simulink model "ACCBase001"  (Simulink 8.3)
settings: Solver=FixedStepDiscrete  StartTime=0.0  StopTime=10.0  FixedStep=0.1  RelTol=1e-3
model workspace (MAT data in the model file):
  pACC.Kp = 0.1
  pACC.minDist2Target = 50
  pACC.Ki = 0.0001
  pACC.KpDist = 1
  pACC.KiDist = 0.0001
  MPS_ModuleName = 'ACC_Enhancement.ECR'
settings Model: Creator=swami  LastModifiedBy=swami
settings DataIOCC: SignalLoggingSaveFormat=Dataset
settings DebuggingCC: UnderspecifiedInitializationDetection=Simplified  StateNameClashWarn=none
settings GRTTargetCC: CombineOutputUpdateFcns=on  GRTInterface=off

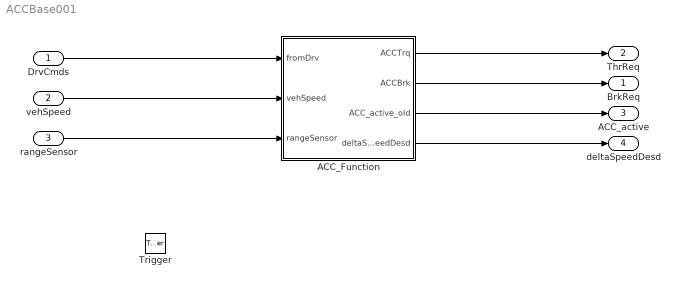
== system ACCBase001 ==
  DrvCmds : Inport  PortDimensions=4
  vehSpeed : Inport  Port=2
  rangeSensor : Inport  Port=3
  Trigger : TriggerPort  TriggerType=function-call  PortDimensions=1
  ACC_Function : MATLAB Function  TreatAsAtomicUnit=on
  BrkReq : Outport  PortDimensions=1
  ThrReq : Outport  Port=2  PortDimensions=1
  ACC_active : Outport  Port=3  PortDimensions=1
  deltaSpeedDesd : Outport  Port=4  PortDimensions=1
  wires:
  DrvCmds/1 -> ACC_Function/1(fromDrv)
  ACC_Function/1(ACCTrq) -> ThrReq/1
  ACC_Function/2(ACCBrk) -> BrkReq/1
  rangeSensor/1 -> ACC_Function/3(rangeSensor)
  vehSpeed/1 -> ACC_Function/2(vehSpeed)
  ACC_Function/3(ACC_active_old) -> ACC_active/1
  ACC_Function/4(deltaSpeedDesd) -> deltaSpeedDesd/1

== matlab function ACC_Function ==
  data: fromDrv input double; ACCTrq output double; ACCBrk output double; vehSpeed input double; rangeSensor input double; pACC parameter double; ACC_active_old output double; deltaSpeedDesd output double
function [ACCTrq,ACCBrk,ACC_active_old,deltaSpeedDesd] = fcn(fromDrv,vehSpeed,rangeSensor,pACC)
%#codegen
persistent dbgcnt;
persistent CC_active;
persistent ACC_active;
persistent torq_req_int;
persistent torq_req_old;
persistent errorKiDist;
if isempty(ACC_active)
    CC_active = 0;
    ACC_active = 0;
    torq_req_int = 0;
    torq_req_old = 0;
    dbgcnt = 0;
    errorKiDist = 0;
end
dbgcnt = dbgcnt + 1;
CC_active_old = CC_active;
ACC_active_old = ACC_active;

deltaSpeedDesd = 0;

DrvBrk = fromDrv(1);
DrvThr = fromDrv(2);
DrvCCSw = fromDrv(3);
DrvCCSetPoint = fromDrv(4);

dist2Target = rangeSensor(1);

minDist2Target = pACC.minDist2Target;
ACCBuffer = minDist2Target * 0.9;

if DrvCCSw > 0.5
    if (CC_active == 0)
        CC_active = 1;
    end
    if (dist2Target < minDist2Target)
        % need to slow down
        ACC_active = 1;
    elseif (dist2Target > (minDist2Target + ACCBuffer))
        ACC_active = 0;
    end
    
    if (ACC_active == 1)            
        errorKpDist = (dist2Target - minDist2Target) * pACC.KpDist;
        errorKiDist = errorKiDist + errorKpDist * pACC.KiDist;
        deltaSpeedDesd = errorKpDist + errorKiDist;
        if deltaSpeedDesd > 0.0
            deltaSpeedDesd = 0;
            ACC_active = 0;
        end
    else
        deltaSpeedDesd = 0;
    end
    
   errorKp = (DrvCCSetPoint +deltaSpeedDesd - vehSpeed) * pACC.Kp;
   
   torq_req_int = torq_req_int + errorKp * pACC.Ki;    
   torq_req_prop = errorKp;   
   torq_req = torq_req_prop + torq_req_int;
   
   if (torq_req > 1.0)
       torq_req = 1.0;
   elseif (torq_req < -1.0)
       torq_req = -1.0;
   end    
   if torq_req < 0.0
       ACCBrk = 0.0 - torq_req;
       ACCTrq = 0.0;
   else
       ACCBrk = 0.0;
       ACCTrq = torq_req;
   end
else
    CC_active = 0;
    ACCTrq = DrvThr;
    ACCBrk = DrvBrk;
    torq_req = ACCTrq;
end
if ((CC_active_old ==0) && (CC_active == 1))
    torq_req_int = torq_req_old;
end

if ((ACC_active_old ==0) && (ACC_active == 1))
    errorKiDist = 0;
    torq_req_int = torq_req_old;
end

torq_req_old = torq_req;
